simulink model "Position_MPC_Adaptive_InnerLoop"  (R2018a)
settings: Solver=VariableStepAuto  StartTime=0.0  StopTime=inf  RelTol=1e-3
undefined symbols (not defined in the file): Ad, Bd, Beta, C1, C2, cBW, d, Discrete, dw, I, Iw, Kb, Kg, Kt, L, La, mc, md, R, Ra, sampleTime, Time, Waypoint
libraries: mobileRoboticsLib x2, cstblocks x2, mpclib x1, ctrlSharedLib x1, dspsrcs4 x1
settings Model: Creator=shravan  LastModifiedBy=shravan

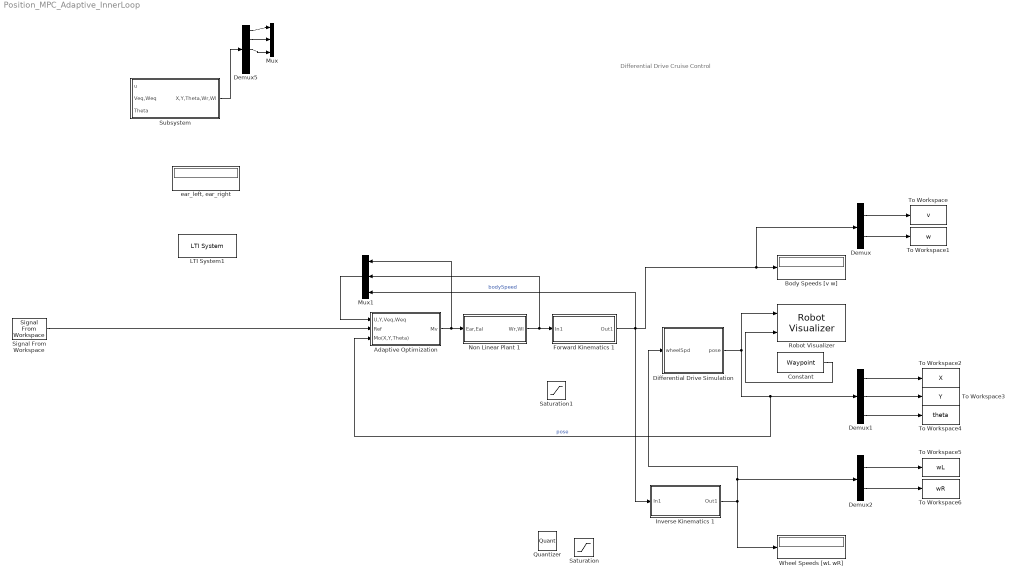
== system Position_MPC_Adaptive_InnerLoop ==
  note: Differential Drive Cruise Control
  "Adaptive Optimization " : Subsystem
  Body Speeds [v w] : Display
  Constant : Constant  Value=Waypoint  SampleTime=sampleTime
  Demux : Demux  Outputs=2
  Demux1 : Demux  Outputs=3
  Demux2 : Demux  Outputs=2
  Demux5 : Demux  Outputs=5
  Differential Drive Simulation : Subsystem  AncestorBlock=mobileRoboticsLib/Kinematic Models/Differential Drive/Differential Drive Simulation  OverrideUsingVariant=mode==2  mask(Differential Drive Simulation){wheelRadius=R, wheelBase=L, initX=C1, initY=C2, initAngle=0, Ts=sampleTime}
      mask prompts: wheelRadius "Wheel Radius [m]"; wheelBase "Wheelbase [m]"; initX "Initial X Position [m]"; initY "Initial Y Position [m]"; initAngle "Initial Angle [rad]"; Ts "Sample Time"
      mask help:
      | Simulates the kinematics of a differential drive vehicle from a specified initial pose.
      |
      | Input: Left and right wheel speeds [wL; wR], in rad/s
      |
      | Output: Pose [x; y; theta], in m, m, and rad
      |
      | Set the Sample Time parameter to 0 for continuous-time simulation, or a positive number for discrete-time simulation.
      mask Help: web('matlab:edit mrsDocDifferentialDrive')
      mask Callback Ts:
      | Ts = evalin('base',get_param(gcb,'Ts'));
      | blk = [gcb '/Generic Robot Simulation/Velocity Integrator'];
      | if Ts > 0
      |     set_param(blk,'OverrideUsingVariant','mode==2');
      | else
      |     set_param(blk,'OverrideUsingVariant','mode==1');
      | end
  Forward Kinematics 1 : Subsystem
  Inverse Kinematics 1 : Subsystem
  LTI System1 : cstblocks/LTI System  sys=Controller  IC=[]
  Mux : Mux  Inputs=3
  Mux1 : Mux  Inputs=3
  Non Linear Plant 1 : Subsystem
  Quantizer : Quantizer
  Robot Visualizer : mobileRoboticsLib/Environments/Robot Visualizer  Priority=99  robotRadius=1  showTrajectory=on  hasWaypoints=on  hasLidar=off  sensorOffset=[ 0 0 ]  scanAngles=[-pi/4,0,pi/4]  hasObjDetector=off  objDetectorOffset=[ 0, 0 ]  objDetectorAngle=0  objDetectorFOV=pi/4  objDetectorMaxRange=5  objectColors=[ 1, 0, 0; 0, 1, 0; 0, 0, 1 ]  objectMarkers='s'
      settings: SourceProductName=Mobile Robotics Simulation Library
  Saturation : Saturate
  Saturation1 : Saturate  UpperLimit=12  LowerLimit=0
  Signal From Workspace : dspsrcs4/Signal From Workspace  X=Lyapunov  Ts=cBW  nsamps=1  OutputAfterFinalValue=Holding final value  ignoreOrWarnInputAndFrameLengths=off  OutputFrames=off
  Subsystem : Subsystem
  To Workspace : ToWorkspace  VariableName=v  SampleTime=-1
  To Workspace1 : ToWorkspace  VariableName=w  SampleTime=-1
  To Workspace2 : ToWorkspace  VariableName=X  SampleTime=sampleTime
  To Workspace3 : ToWorkspace  VariableName=Y  SampleTime=-1
  To Workspace4 : ToWorkspace  VariableName=theta  SampleTime=-1
  To Workspace5 : ToWorkspace  VariableName=wL  SampleTime=-1
  To Workspace6 : ToWorkspace  VariableName=wR  SampleTime=-1
  Wheel Speeds [wL wR] : Display
  "ear_left, ear_right " : Display
  wires:
  Demux5/2 -> Mux/2
  Subsystem/1(X,Y,Theta,Wr,Wl) -> Demux5/1
  Demux5/1 -> Mux/1
  Demux5/3 -> Mux/3
  Inverse Kinematics 1/1(Out1) -> Differential Drive Simulation/1(wheelSpd), Demux2/1, Wheel Speeds [wL wR]/1
  Demux2/2 -> To Workspace6/1
  Demux1/3 -> To Workspace4/1
  Demux1/2 -> To Workspace3/1
  Demux/1 -> To Workspace/1
  Demux/2 -> To Workspace1/1
  "Adaptive Optimization "/1(Mv) -> Non Linear Plant 1/1("Ear,Eal "), Mux1/1
  Differential Drive Simulation/1(pose) -> "Adaptive Optimization "/3(Mo(X,Y,Theta)), Demux1/1, Robot Visualizer/1  "pose"
  Non Linear Plant 1/1(Wr,Wl) -> Mux1/2, Forward Kinematics 1/1(In1)
  Demux1/1 -> To Workspace2/1
  Mux1/1 -> "Adaptive Optimization "/1(U,Y,Veq,Weq)
  Demux2/1 -> To Workspace5/1
  Constant/1 -> Robot Visualizer/2
  Forward Kinematics 1/1(Out1) -> Mux1/3, Inverse Kinematics 1/1(In1), Demux/1, Body Speeds [v w]/1  "bodySpeed"
  Signal From Workspace/1 -> "Adaptive Optimization "/2(Ref)

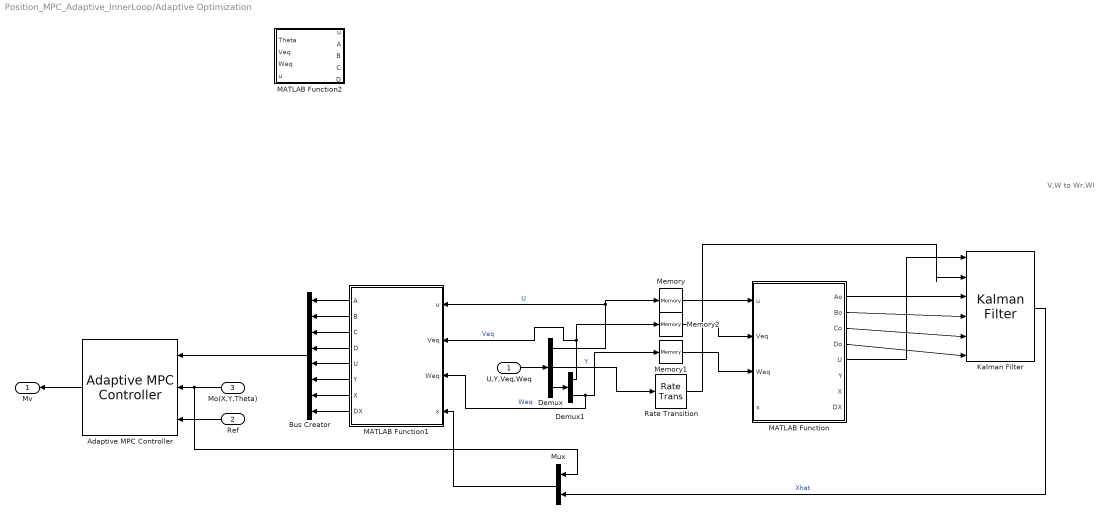
== system Position_MPC_Adaptive_InnerLoop/Adaptive Optimization  ==
  note: V,W to Wr,Wl
  U,Y,Veq,Weq : Inport
  Ref : Inport  Port=2
  Mo(X,Y,Theta) : Inport  Port=3
  Adaptive MPC Controller : mpclib/Adaptive MPC Controller  SCDEnableBlockLinearizationSpecification=on  mpcobj=mpc_pos  updateMPCinCallerWorkspace=on  md_inport=off  mv_inport=off  cost_outport=off  return_sequence=off  return_qpstatus=off  return_state=off  state_inport=off  isltv_plant=off  lims_inport=off  cc_inport=off  ywt_inport=off  uwt_inport=off  duwt_inport=off  rhoeps_inport=off  uref_inport=off  BlockDataType=double  SampleTimeInherited=off  switch_inport=off
      settings: SourceProductName=Model Predictive Control Toolbox
  Bus Creator : BusCreator  Inputs=8
  Demux : Demux  Outputs=3
  Demux1 : Demux  Outputs=2
  Kalman Filter : ctrlSharedLib/Kalman Filter  TimeDomain=Discrete-Time  UseCurrentEstimator=on  ModelSource=Input port  ModelSourceVariable=Plant  A=0.95  B=1  C=1  D=0  NumberOfStates=4  NumberOfInputs=2  NumberOfOutputs=2  InitialEstimateSource=Dialog  X0=0  P0=0.1  UseK=off  UseGH=off  NumberOfProcessNoiseInputs=1  G=1  TimeInvariantG=on  H=0  TimeInvariantH=on  Q=diag([100 100 100 100])  TimeInvariantQ=on  R=diag([0.0001 0.0001])  TimeInvariantR=on  N=0  TimeInvariantN=on  AddInputPort=on  AddEnablePort=off  OutputEstimatedY=off  OutputP=off  Ts=sampleTime
      settings: SourceProductBaseCode=CT
  MATLAB Function : MATLAB Function  TreatAsAtomicUnit=on  SystemSampleTime=sampleTime
  MATLAB Function1 : MATLAB Function  TreatAsAtomicUnit=on  SystemSampleTime=sampleTime
  MATLAB Function2 : MATLAB Function  TreatAsAtomicUnit=on  SystemSampleTime=sampleTime*0.1
  Memory : Memory
  Memory1 : Memory
  Memory2 : Memory
  Mux : Mux  Inputs=2
  Rate Transition : RateTransition  OutPortSampleTime=sampleTime
  Mv : Outport
  wires:
  U,Y,Veq,Weq/1 -> Demux/1
  Memory/1 -> MATLAB Function/1(u)
  Demux/1 -> Memory/1, MATLAB Function1/1(u)  "U"
  Memory2/1 -> MATLAB Function/2(Veq)
  Memory1/1 -> MATLAB Function/3(Weq)
  MATLAB Function/1(Ao) -> Kalman Filter/3
  MATLAB Function/2(Bo) -> Kalman Filter/4
  MATLAB Function/3(Co) -> Kalman Filter/5
  MATLAB Function/4(Do) -> Kalman Filter/6
  MATLAB Function/5(U) -> Kalman Filter/1
  Demux/2 -> Rate Transition/1  "Y"
  Rate Transition/1 -> Kalman Filter/2
  MATLAB Function1/1(A) -> Bus Creator/1
  MATLAB Function1/2(B) -> Bus Creator/2
  MATLAB Function1/3(C) -> Bus Creator/3
  MATLAB Function1/4(D) -> Bus Creator/4
  MATLAB Function1/5(U) -> Bus Creator/5
  MATLAB Function1/6(Y) -> Bus Creator/6
  MATLAB Function1/7(X) -> Bus Creator/7
  MATLAB Function1/8(DX) -> Bus Creator/8
  Bus Creator/1 -> Adaptive MPC Controller/1
  Mo(X,Y,Theta)/1 -> Mux/1, Adaptive MPC Controller/2
  Ref/1 -> Adaptive MPC Controller/3
  Adaptive MPC Controller/1 -> Mv/1
  Demux/3 -> Demux1/1
  Demux1/1 -> MATLAB Function1/2(Veq), Memory2/1  "Veq"
  Demux1/2 -> MATLAB Function1/3(Weq), Memory1/1  "Weq"
  Kalman Filter/1 -> Mux/2  "Xhat"
  Mux/1 -> MATLAB Function1/4(x)

== system Position_MPC_Adaptive_InnerLoop/Differential Drive Simulation ==
  wheelSpd : Inport
  Constant : Constant  Value=0
  Demux : Demux  Outputs=2
  Forward Kinematics 1 : Subsystem
  Generic Robot Simulation : mobileRoboticsLib/Utilities/Generic Vehicle Simulation  initX=initX  initY=initY  initAngle=initAngle  Ts=Ts
      link override Velocity Integrator: OverrideUsingVariant=mode==2
      settings: SourceProductName=Mobile Robotics Simulation Toolbox
  Mux1 : Mux  Inputs=3
  pose : Outport
  wires:
  Generic Robot Simulation/1 -> pose/1
  Forward Kinematics 1/1(Out1) -> Demux/1
  wheelSpd/1 -> Forward Kinematics 1/1(In1)
  Constant/1 -> Mux1/2  "vy"
  Demux/2 -> Mux1/3  "w"
  Demux/1 -> Mux1/1  "vx"
  Mux1/1 -> Generic Robot Simulation/1

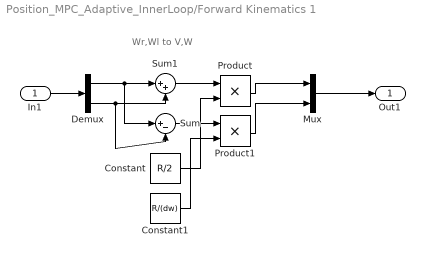
== system Position_MPC_Adaptive_InnerLoop/Forward Kinematics 1 ==
  note: Wr,Wl to V,W
  In1 : Inport
  Constant : Constant  Value=R/2
  Constant1 : Constant  Value=R/(dw)
  Demux : Demux  Outputs=2
  Mux : Mux  Inputs=2
  Product : Product
  Product1 : Product
  Sum : Sum  Inputs=|+-
  Sum1 : Sum  Inputs=|++
  Out1 : Outport
  wires:
  In1/1 -> Demux/1
  Product1/1 -> Mux/2
  Mux/1 -> Out1/1
  Product/1 -> Mux/1
  Demux/1 -> Sum/1, Sum1/1
  Demux/2 -> Sum/2, Sum1/2
  Sum1/1 -> Product/1
  Constant/1 -> Product/2
  Sum/1 -> Product1/1
  Constant1/1 -> Product1/2

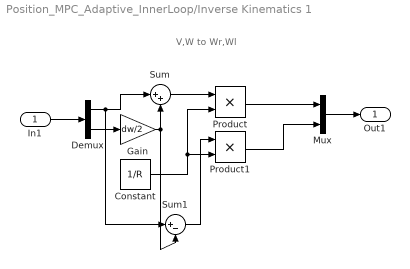
== system Position_MPC_Adaptive_InnerLoop/Inverse Kinematics 1 ==
  note: V,W to Wr,Wl
  In1 : Inport
  Constant : Constant  Value=1/R
  Demux : Demux  Outputs=2
  Gain : Gain  Gain=dw/2
  Mux : Mux  Inputs=2
  Product : Product
  Product1 : Product
  Sum : Sum  Inputs=|++
  Sum1 : Sum  Inputs=|+-
  Out1 : Outport
  wires:
  Gain/1 -> Sum/2, Sum1/2
  Product1/1 -> Mux/2
  Product/1 -> Mux/1
  Sum1/1 -> Product1/1
  Constant/1 -> Product/2, Product1/2
  Sum/1 -> Product/1
  Demux/1 -> Sum/1, Sum1/1
  Demux/2 -> Gain/1
  In1/1 -> Demux/1
  Mux/1 -> Out1/1

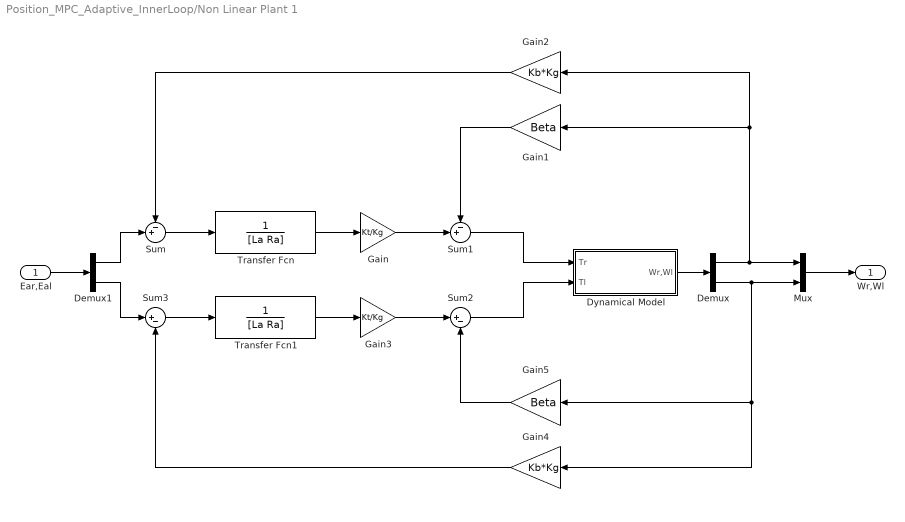
== system Position_MPC_Adaptive_InnerLoop/Non Linear Plant 1 ==
  "Ear,Eal " : Inport
  Demux : Demux  Outputs=2
  Demux1 : Demux  Outputs=2
  Dynamical Model : Subsystem
  Gain : Gain  Gain=Kt/Kg
  Gain1 : Gain  Gain=Beta
  Gain2 : Gain  Gain=Kb*Kg
  Gain3 : Gain  Gain=Kt/Kg
  Gain4 : Gain  Gain=Kb*Kg
  Gain5 : Gain  Gain=Beta
  Mux : Mux  Inputs=2
  Sum : Sum  Inputs=-+|
  Sum1 : Sum  Inputs=-+|
  Sum2 : Sum  Inputs=|+-
  Sum3 : Sum  Inputs=|+-
  Transfer Fcn : TransferFcn  Denominator=[La Ra]
  Transfer Fcn1 : TransferFcn  Denominator=[La Ra]
  Wr,Wl : Outport
  wires:
  Sum2/1 -> Dynamical Model/2(Tl)
  Demux/2 -> Mux/2, Gain5/1, Gain4/1
  Gain3/1 -> Sum2/1
  Transfer Fcn1/1 -> Gain3/1
  Transfer Fcn/1 -> Gain/1
  Sum1/1 -> Dynamical Model/1(Tr)
  "Ear,Eal "/1 -> Demux1/1
  Gain/1 -> Sum1/2
  Gain2/1 -> Sum/1
  Mux/1 -> Wr,Wl/1
  Sum3/1 -> Transfer Fcn1/1
  Demux1/1 -> Sum/2
  Dynamical Model/1(Wr,Wl) -> Demux/1
  Demux/1 -> Gain1/1, Gain2/1, Mux/1
  Gain1/1 -> Sum1/1
  Demux1/2 -> Sum3/1
  Sum/1 -> Transfer Fcn/1
  Gain4/1 -> Sum3/2
  Gain5/1 -> Sum2/2

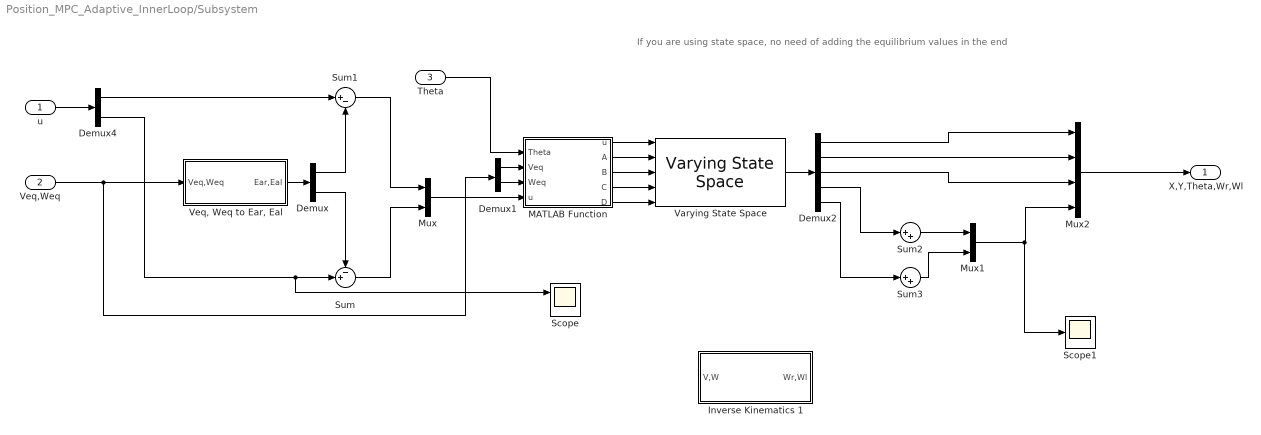
== system Position_MPC_Adaptive_InnerLoop/Subsystem ==
  note: If you are using state space, no need of adding the equilibrium values in the end
  "u " : Inport
  "Veq,Weq " : Inport  Port=2
  "Theta " : Inport  Port=3
  Demux : Demux  Outputs=2
  Demux1 : Demux  Outputs=2
  Demux2 : Demux  Outputs=5
  Demux4 : Demux  Outputs=2
  Inverse Kinematics 1 : Subsystem
  MATLAB Function : MATLAB Function  TreatAsAtomicUnit=on  SystemSampleTime=sampleTime*0.1
  Mux : Mux  Inputs=2
  Mux1 : Mux  Inputs=2
  Mux2 : Mux
  Scope : Scope  NumInputPorts=2
  Scope1 : Scope
  Sum : Sum  Inputs=-+|
  Sum1 : Sum  Inputs=|+-
  Sum2 : Sum  Inputs=|++
  Sum3 : Sum  Inputs=|++
  Varying State Space : cstblocks/Linear Parameter Varying/Varying State Space  x0=[C1;C2;0;0;0;0;0]  xNames=''  OutputX=off  OutputDX=off
      settings: SourceProductName=Control System Toolbox
  "Veq, Weq to Ear, Eal " : Subsystem
  X,Y,Theta,Wr,Wl : Outport
  wires:
  "Veq, Weq to Ear, Eal "/1(Ear,Eal) -> Demux/1
  Demux/1 -> Sum1/2
  Demux/2 -> Sum/1
  MATLAB Function/3(B) -> Varying State Space/3
  MATLAB Function/4(C) -> Varying State Space/4
  MATLAB Function/1(u) -> Varying State Space/1
  MATLAB Function/2(A) -> Varying State Space/2
  MATLAB Function/5(D) -> Varying State Space/5
  Sum1/1 -> Mux/1
  Sum/1 -> Mux/2
  Mux/1 -> MATLAB Function/4("u ")
  "Theta "/1 -> MATLAB Function/1(Theta)
  Demux1/2 -> MATLAB Function/3(Weq)
  Demux1/1 -> MATLAB Function/2(Veq)
  Varying State Space/1 -> Demux2/1
  Demux2/1 -> Mux2/1
  Demux2/2 -> Mux2/2
  Demux2/3 -> Mux2/3
  Demux2/4 -> Sum2/1
  Demux2/5 -> Sum3/1
  Mux1/1 -> Scope1/1, Mux2/4
  Sum2/1 -> Mux1/1
  Sum3/1 -> Mux1/2
  "Veq,Weq "/1 -> "Veq, Weq to Ear, Eal "/1(Veq,Weq), Demux1/1
  Mux2/1 -> X,Y,Theta,Wr,Wl/1
  "u "/1 -> Demux4/1
  Demux4/1 -> Sum1/1
  Demux4/2 -> Scope/1, Sum/2

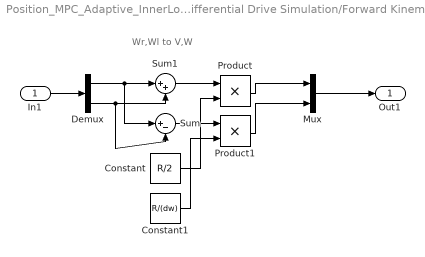
== system Position_MPC_Adaptive_InnerLoop/Differential Drive Simulation/Forward Kinematics 1 ==
  note: Wr,Wl to V,W
  In1 : Inport
  Constant : Constant  Value=R/2
  Constant1 : Constant  Value=R/(dw)
  Demux : Demux  Outputs=2
  Mux : Mux  Inputs=2
  Product : Product
  Product1 : Product
  Sum : Sum  Inputs=|+-
  Sum1 : Sum  Inputs=|++
  Out1 : Outport
  wires:
  In1/1 -> Demux/1
  Product1/1 -> Mux/2
  Mux/1 -> Out1/1
  Product/1 -> Mux/1
  Demux/1 -> Sum/1, Sum1/1
  Demux/2 -> Sum/2, Sum1/2
  Sum1/1 -> Product/1
  Constant/1 -> Product/2
  Sum/1 -> Product1/1
  Constant1/1 -> Product1/2

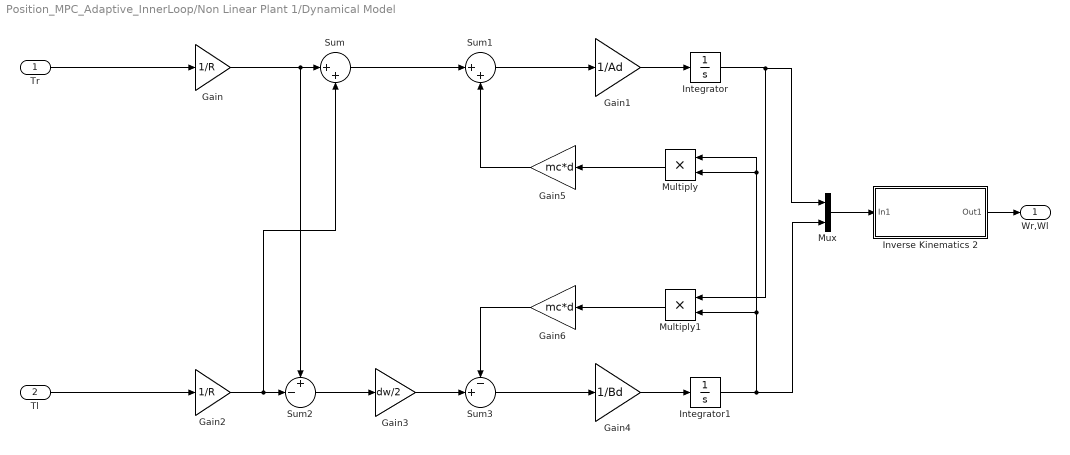
== system Position_MPC_Adaptive_InnerLoop/Non Linear Plant 1/Dynamical Model ==
  Tr : Inport
  Tl : Inport  Port=2
  Gain : Gain  Gain=1/R
  Gain1 : Gain  Gain=1/Ad
  Gain2 : Gain  Gain=1/R
  Gain3 : Gain  Gain=dw/2
  Gain4 : Gain  Gain=1/Bd
  Gain5 : Gain  Gain=mc*d
  Gain6 : Gain  Gain=mc*d
  Integrator : Integrator
  Integrator1 : Integrator
  Inverse Kinematics 2 : Subsystem
  Multiply : Product
  Multiply1 : Product
  Mux : Mux  Inputs=2
  Sum : Sum  Inputs=|++
  Sum1 : Sum  Inputs=|++
  Sum2 : Sum  Inputs=+-|
  Sum3 : Sum  Inputs=-+|
  Wr,Wl : Outport
  wires:
  Gain1/1 -> Integrator/1
  Tl/1 -> Gain2/1
  Gain6/1 -> Sum3/1
  Gain2/1 -> Sum2/2, Sum/2
  Sum2/1 -> Gain3/1
  Gain3/1 -> Sum3/2
  Multiply/1 -> Gain5/1
  Integrator1/1 -> Mux/2, Multiply/1, Multiply/2, Multiply1/2
  Tr/1 -> Gain/1
  Gain5/1 -> Sum1/2
  Sum/1 -> Sum1/1
  Inverse Kinematics 2/1(Out1) -> Wr,Wl/1
  Gain4/1 -> Integrator1/1
  Mux/1 -> Inverse Kinematics 2/1(In1)
  Integrator/1 -> Multiply1/1, Mux/1
  Gain/1 -> Sum2/1, Sum/1
  Sum3/1 -> Gain4/1
  Multiply1/1 -> Gain6/1
  Sum1/1 -> Gain1/1

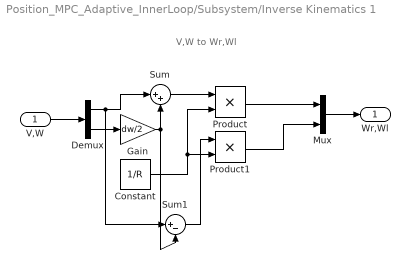
== system Position_MPC_Adaptive_InnerLoop/Subsystem/Inverse Kinematics 1 ==
  note: V,W to Wr,Wl
  V,W : Inport
  Constant : Constant  Value=1/R
  Demux : Demux  Outputs=2
  Gain : Gain  Gain=dw/2
  Mux : Mux  Inputs=2
  Product : Product
  Product1 : Product
  Sum : Sum  Inputs=|++
  Sum1 : Sum  Inputs=|+-
  Wr,Wl : Outport
  wires:
  Gain/1 -> Sum/2, Sum1/2
  Product1/1 -> Mux/2
  Product/1 -> Mux/1
  Sum1/1 -> Product1/1
  Constant/1 -> Product/2, Product1/2
  Sum/1 -> Product/1
  Demux/1 -> Sum/1, Sum1/1
  Demux/2 -> Gain/1
  V,W/1 -> Demux/1
  Mux/1 -> Wr,Wl/1

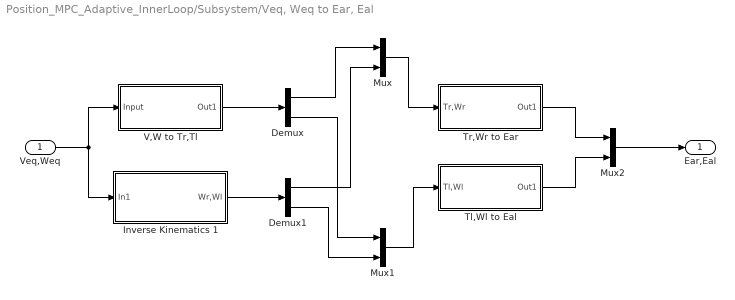
== system Position_MPC_Adaptive_InnerLoop/Subsystem/Veq, Weq to Ear, Eal  ==
  Veq,Weq : Inport
  Demux : Demux  Outputs=2
  Demux1 : Demux  Outputs=2
  Inverse Kinematics 1 : Subsystem
  Mux : Mux  Inputs=2
  Mux1 : Mux  Inputs=2
  Mux2 : Mux  Inputs=2
  Tl,Wl to Eal : Subsystem
  Tr,Wr to Ear : Subsystem
  V,W to Tr,Tl : Subsystem
  Ear,Eal : Outport
  wires:
  V,W to Tr,Tl/1(Out1) -> Demux/1
  Demux/1 -> Mux/1
  Mux/1 -> Tr,Wr to Ear/1(Tr,Wr)
  Veq,Weq/1 -> Inverse Kinematics 1/1(In1), V,W to Tr,Tl/1(Input)
  Inverse Kinematics 1/1(Wr,Wl) -> Demux1/1
  Demux1/1 -> Mux/2
  Demux/2 -> Mux1/1
  Demux1/2 -> Mux1/2
  Mux1/1 -> Tl,Wl to Eal/1(Tl,Wl)
  Tr,Wr to Ear/1(Out1) -> Mux2/1
  Tl,Wl to Eal/1(Out1) -> Mux2/2
  Mux2/1 -> Ear,Eal/1

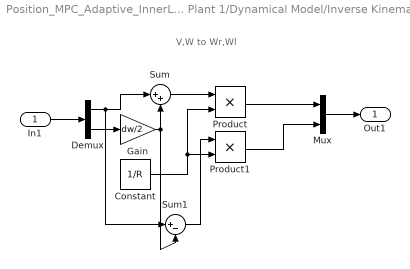
== system Position_MPC_Adaptive_InnerLoop/Non Linear Plant 1/Dynamical Model/Inverse Kinematics 2 ==
  note: V,W to Wr,Wl
  In1 : Inport
  Constant : Constant  Value=1/R
  Demux : Demux  Outputs=2
  Gain : Gain  Gain=dw/2
  Mux : Mux  Inputs=2
  Product : Product
  Product1 : Product
  Sum : Sum  Inputs=|++
  Sum1 : Sum  Inputs=|+-
  Out1 : Outport
  wires:
  Product1/1 -> Mux/2
  Product/1 -> Mux/1
  Sum1/1 -> Product1/1
  Constant/1 -> Product/2, Product1/2
  Sum/1 -> Product/1
  Gain/1 -> Sum/2, Sum1/2
  Demux/1 -> Sum/1, Sum1/1
  Demux/2 -> Gain/1
  In1/1 -> Demux/1
  Mux/1 -> Out1/1

== system Position_MPC_Adaptive_InnerLoop/Subsystem/Veq, Weq to Ear, Eal /Inverse Kinematics 1 ==
  note: V,W to Wr,Wl
  In1 : Inport
  Constant : Constant  Value=1/R
  Demux : Demux  Outputs=2
  Gain : Gain  Gain=dw/2
  Mux : Mux  Inputs=2
  Product : Product
  Product1 : Product
  Sum : Sum  Inputs=|++
  Sum1 : Sum  Inputs=|+-
  Wr,Wl : Outport
  wires:
  Mux/1 -> Wr,Wl/1
  In1/1 -> Demux/1
  Demux/2 -> Gain/1
  Demux/1 -> Sum1/1, Sum/1
  Sum/1 -> Product/1
  Constant/1 -> Product1/2, Product/2
  Sum1/1 -> Product1/1
  Product/1 -> Mux/1
  Product1/1 -> Mux/2
  Gain/1 -> Sum1/2, Sum/2

== system Position_MPC_Adaptive_InnerLoop/Subsystem/Veq, Weq to Ear, Eal /Tl,Wl to Eal ==
  Tl,Wl : Inport
  Demux1 : Demux  Outputs=2
  Gain : Gain  Gain=Ra*Kg/Kt
  Gain1 : Gain  Gain=Beta
  Gain2 : Gain  Gain=Ra*Kg/Kt
  Gain3 : Gain  Gain=Kb*Kg
  Sum : Sum  Inputs=|+++
  Out1 : Outport
  wires:
  Gain1/1 -> Sum/2
  Gain2/1 -> Gain1/1
  Gain/1 -> Sum/1
  Gain3/1 -> Sum/3
  Sum/1 -> Out1/1
  Tl,Wl/1 -> Demux1/1
  Demux1/1 -> Gain/1
  Demux1/2 -> Gain3/1, Gain2/1

== system Position_MPC_Adaptive_InnerLoop/Subsystem/Veq, Weq to Ear, Eal /Tr,Wr to Ear ==
  Tr,Wr : Inport
  Demux1 : Demux  Outputs=2
  Gain : Gain  Gain=Ra*Kg/Kt
  Gain1 : Gain  Gain=Beta
  Gain2 : Gain  Gain=Ra*Kg/Kt
  Gain3 : Gain  Gain=Kb*Kg
  Sum : Sum  Inputs=|+++
  Out1 : Outport
  wires:
  Gain2/1 -> Gain1/1
  Tr,Wr/1 -> Demux1/1
  Sum/1 -> Out1/1
  Gain1/1 -> Sum/2
  Gain3/1 -> Sum/3
  Demux1/2 -> Gain3/1, Gain2/1
  Gain/1 -> Sum/1
  Demux1/1 -> Gain/1

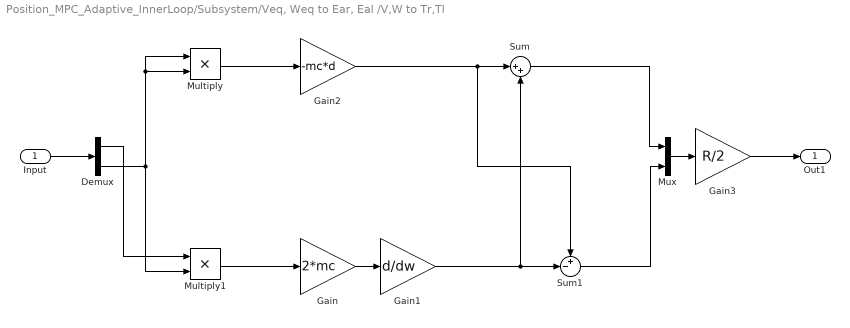
== system Position_MPC_Adaptive_InnerLoop/Subsystem/Veq, Weq to Ear, Eal /V,W to Tr,Tl ==
  Input : Inport
  Demux : Demux  Outputs=2
  Gain : Gain  Gain=2*mc
  Gain1 : Gain  Gain=d/dw
  Gain2 : Gain  Gain=-mc*d
  Gain3 : Gain  Gain=R/2
  Multiply : Product
  Multiply1 : Product
  Mux : Mux  Inputs=2
  Sum : Sum  Inputs=|++
  Sum1 : Sum  Inputs=+-|
  Out1 : Outport
  wires:
  Demux/1 -> Multiply1/1
  Mux/1 -> Gain3/1
  Gain/1 -> Gain1/1
  Input/1 -> Demux/1
  Multiply1/1 -> Gain/1
  Sum1/1 -> Mux/2
  Gain1/1 -> Sum1/2, Sum/2
  Gain2/1 -> Sum1/1, Sum/1
  Demux/2 -> Multiply1/2, Multiply/2, Multiply/1
  Gain3/1 -> Out1/1
  Multiply/1 -> Gain2/1
  Sum/1 -> Mux/1

== matlab function Position_MPC_Adaptive_InnerLoop/Adaptive Optimization /MATLAB Function2 ==
  data: Theta input size=[1,1]; Veq input size=[1,1]; Weq input size=[1,1]; u input size=[2,1]; u output; A output; B output; C output; D output; sampleTime parameter; I parameter; Iw parameter; R parameter
function [u,A,B,C,D] = fcn(Theta,Veq,Weq,u,sampleTime,I, Iw,R)
% Sample time
Ts = sampleTime;
d = 0.0107; L = 0.28; AR = L/0.25; dw = 0.25; md = 0;
d = 0; thetaeq = Theta;
% Model Parameters
Kt = 0.0046; Kg = 50; Kb = Kt; Beta = 2.29e-06; La =1.729e-03; Ra = 5.51;
m = 3.4; mc = 2.76 + md; I = I ; Iw = Iw; L = L; d = d; dw = dw; 
Ao = m + 2*Iw/(R*R); Bo = I + dw*dw*Iw/(2*R*R);

% Continuous-time model for Plant e_r, e_l to Wr,Wl
% ULTIMATE - CORRECT representation of Plant using State Space form derived
% on Aug 24 th, 2020 
Ac = [-2*Beta/(Ao*R*R) 2*mc*d*Weq/Ao   (Kt/(Kg*R*Ao))  (Kt/(Kg*R*Ao));
     -mc*d*Weq/Bo  (-mc*d*Veq/Bo)-(Beta*dw*dw/(2*R*R*Bo)) dw*Kt/(2*Kg*R*Bo) -dw*Kt/(2*Kg*Bo*R) ;
     -Kb*Kg/(La*R)   -Kb*Kg*dw/(2*La*R)  -Ra/La      0 ;
     -Kb*Kg/(La*R)    Kb*Kg*dw/(2*La*R)    0       -Ra/La ];
Bc = [0 0; 0 0; 1/La 0; 0 1/La]; Cc =  [1/R dw/(2*R); 1/R -dw/(2*R)]*[1 0 0 0; 0 1 0 0]; Dc = [0 0;0 0];


% States x,y,theta, V,W, Iar,Ial 

Au =      [0  0  -Veq*sin(thetaeq) cos(thetaeq)  0  0  0;
           0  0  Veq*cos(thetaeq) sin(thetaeq)  0  0  0;
           0  0  0                 0            1  0  0;  
           zeros(4,3) Ac]
Bu =      [0 0;
           0 0;
           0 0;
           Bc]
Cu =      [1 0 0 0 0 0 0;
           0 1 0 0 0 0 0;
           0 0 1 0 0 0 0;
           zeros(2,3) Cc]
Du =       zeros(5,2)

% Discretize the continuous-time model using zero-order hold 
% on the inputs and a sample time of Ts seconds
nx = size(Au,1);
nu = size(Bu,2);
M = expm([[Au Bu]*Ts; zeros(nu,nx+nu)]);
A = Au;%M(1:nx,1:nx);
B = Bu;%M(1:nx,nx+1:nx+nu);
C = Cu;
D = Du;

% Nominal conditions for discrete-time plant
%X = x;
u = u;
%Y = Co*x + Do*u;
%DX = Ao*x+Bo*u-x;
%y = u;

== matlab function Position_MPC_Adaptive_InnerLoop/Subsystem/MATLAB Function ==
  data: Theta input size=[1,1]; Veq input size=[1,1]; Weq input size=[1,1]; u input size=[2,1]; u output; A output; B output; C output; D output; sampleTime parameter; I parameter; Iw parameter; R parameter
function [u,A,B,C,D] = fcn(Theta,Veq,Weq,u,sampleTime,I, Iw,R)
% Sample time
Ts = sampleTime;
d = 0.0107; L = 0.28; AR = L/0.25; dw = 0.25; md = 0;
d = 0; thetaeq = Theta;
% Model Parameters
Kt = 0.0046; Kg = 50; Kb = Kt; Beta = 2.29e-06; La =1.729e-03; Ra = 5.51;
m = 3.4; mc = 2.76 + md; I = I ; Iw = Iw; L = L; d = d; dw = dw; 
Ao = m + 2*Iw/(R*R); Bo = I + dw*dw*Iw/(2*R*R);

% Continuous-time model for Plant e_r, e_l to Wr,Wl
% ULTIMATE - CORRECT representation of Plant using State Space form derived
% on Aug 24 th, 2020 
Ac = [-2*Beta/(Ao*R*R) 2*mc*d*Weq/Ao   (Kt/(Kg*R*Ao))  (Kt/(Kg*R*Ao));
     -mc*d*Weq/Bo  (-mc*d*Veq/Bo)-(Beta*dw*dw/(2*R*R*Bo)) dw*Kt/(2*Kg*R*Bo) -dw*Kt/(2*Kg*Bo*R) ;
     -Kb*Kg/(La*R)   -Kb*Kg*dw/(2*La*R)  -Ra/La      0 ;
     -Kb*Kg/(La*R)    Kb*Kg*dw/(2*La*R)    0       -Ra/La ];
Bc = [0 0; 0 0; 1/La 0; 0 1/La]; Cc =  [1/R dw/(2*R); 1/R -dw/(2*R)]*[1 0 0 0; 0 1 0 0]; Dc = [0 0;0 0];


% States x,y,theta, V,W, Iar,Ial 

Au =      [0  0  -Veq*sin(thetaeq) cos(thetaeq)  0  0  0;
           0  0  Veq*cos(thetaeq) sin(thetaeq)  0  0  0;
           0  0  0                 0            1  0  0;  
           zeros(4,3) Ac]
Bu =      [0 0;
           0 0;
           0 0;
           Bc]
Cu =      [1 0 0 0 0 0 0;
           0 1 0 0 0 0 0;
           0 0 1 0 0 0 0;
           zeros(2,3) Cc]
Du =       zeros(5,2)

% Discretize the continuous-time model using zero-order hold 
% on the inputs and a sample time of Ts seconds
nx = size(Au,1);
nu = size(Bu,2);
M = expm([[Au Bu]*Ts; zeros(nu,nx+nu)]);
A = Au;%M(1:nx,1:nx);
B = Bu;%M(1:nx,nx+1:nx+nu);
C = Cu;
D = Du;

% Nominal conditions for discrete-time plant
%X = x;
u = u;
%Y = Co*x + Do*u;
%DX = Ao*x+Bo*u-x;
%y = u;

== matlab function Position_MPC_Adaptive_InnerLoop/Adaptive Optimization /MATLAB Function ==
  data: u input size=[2,1]; Veq input size=[1,1]; Weq input size=[1,1]; Ao output size=[4,4]; x input size=[4,1]; Bo output size=[4,2]; Co output size=[2,4]; Do output size=[2,2]; U output size=[2,1]; Y output size=[2,1]; X output size=[4,1]; DX output size=[4,1]; sampleTime parameter size=[1,1]; d parameter size=[1,1]; dw parameter size=[1,1]; Iw parameter size=[1,1]; I parameter size=[1,1]; md parameter size=1,1; R parameter size=1,1; L parameter size=1,1
function [Ao,Bo,Co,Do,U,Y,X,DX] = fcn(u,Veq,Weq,x,sampleTime,d, dw, Iw, I, md, R, L)
% Sample time
Ts = sampleTime;

% Model Parameters
Kt = 0.0046; Kg = 50; Kb = Kt; Beta = 2.29e-06; La =1.729e-03; Ra = 5.51;
m = 3.4; mc = 2.76 + md; I = I ; Iw = Iw; L = L; d = d; dw = dw; 
A = m + 2*Iw/(R*R); B = I + dw*dw*Iw/(2*R*R);

% Continuous-time model for Plant e_r, e_l to Wr,Wl
Ac = [-2*Beta*Kg*Kg/(A*R*R)  2*mc*d*Weq/A   (Kt*Kg/(R*A))  (Kt*Kg/(A*R));
      -mc*d*Weq/B  (-mc*d*Veq/B)-(Beta*dw*dw*Kg*Kg/(2*R*R*B)) dw*Kt*Kg/(2*R*B) -dw*Kt*Kg/(2*B*R) ;
     -Kb*Kg/(La*R)   -Kb*Kg*dw/(2*La*R)  -Ra/La      0 ;
     -Kb*Kg/(La*R)    Kb*Kg*dw/(2*La*R)    0       -Ra/La ];
Bc = [0 0; 0 0; 1/La 0; 0 1/La]; Cc =  [1/R dw/(2*R); 1/R -dw/(2*R)]*[1 0 0 0; 0 1 0 0]; Dc = [0 0;0 0];


% Discretize the continuous-time model using zero-order hold 
% on the inputs and a sample time of Ts seconds
nx = size(Ac,1);
nu = size(Bc,2);
M = expm([[Ac Bc]*Ts; zeros(nu,nx+nu)]);
Ao = M(1:nx,1:nx);
Bo = M(1:nx,nx+1:nx+nu);
Co = Cc;
Do = Dc;

% Nominal conditions for discrete-time plant
X = x;
U = u;
Y = Co*x + Do*u;
DX = Ao*x+Bo*u-x;

== matlab function Position_MPC_Adaptive_InnerLoop/Adaptive Optimization /MATLAB Function1 ==
  data: u input size=[2,1]; Veq input size=[1,1]; Weq input size=[1,1]; A output size=[7,7]; x input size=[7,1]; B output size=[7,2]; C output size=[3,7]; D output size=[3,2]; U output size=[2,1]; Y output size=[3,1]; X output size=[7,1]; DX output size=[7,1]; sampleTime parameter size=[1,1]; d parameter size=[1,1]; dw parameter size=[1,1]; Iw parameter size=[1,1]; I parameter size=[1,1]; md parameter size=1,1; R parameter size=1,1; L parameter size=1,1
function [A,B,C,D,U,Y,X,DX] = fcn(u,Veq,Weq,x,sampleTime,d, dw, Iw, I, md, R, L)
% Sample time
Ts = sampleTime;

% Model Parameters
Kt = 0.0046; Kg = 50; Kb = Kt; Beta = 2.29e-06; La =1.729e-03; Ra = 5.51;
m = 3.4; mc = 2.76 + md; I = I ; Iw = Iw; L = L; d = d; dw = dw; 
Ao = m + 2*Iw/(R*R); Bo = I + dw*dw*Iw/(2*R*R);
thetaeq = x(3,1);
% Continuous-time model for Plant e_r, e_l to Wr,Wl
% ULTIMATE - CORRECT representation of Plant using State Space form derived
% on Aug 24 th, 2020 
Ac = [-2*Beta/(Ao*R*R) 2*mc*d*Weq/Ao   (Kt/(Kg*R*Ao))  (Kt/(Kg*R*Ao));
     -mc*d*Weq/Bo  (-mc*d*Veq/Bo)-(Beta*dw*dw/(2*R*R*Bo)) dw*Kt/(2*Kg*R*Bo) -dw*Kt/(2*Kg*Bo*R) ;
     -Kb*Kg/(La*R)   -Kb*Kg*dw/(2*La*R)  -Ra/La      0 ;
     -Kb*Kg/(La*R)    Kb*Kg*dw/(2*La*R)    0       -Ra/La ];
Bc = [0 0; 0 0; 1/La 0; 0 1/La]; Cc =  [1/R dw/(2*R); 1/R -dw/(2*R)]*[1 0 0 0; 0 1 0 0]; Dc = [0 0;0 0];


% States x,y,theta, V,W, Iar,Ial 

Au =      [0  0  -Veq*sin(thetaeq) cos(thetaeq)  0  0  0;
           0  0  Veq*cos(thetaeq) sin(thetaeq)  0  0  0;
           0  0  0                 0            1  0  0;  
           zeros(4,3) Ac]
Bu =      [0 0;
           0 0;
           0 0;
           Bc]
Cu =      [1 0 0 0 0 0 0;
           0 1 0 0 0 0 0;
           0 0 1 0 0 0 0]
Du =       zeros(3,2)

% Discretize the continuous-time model using zero-order hold 
% on the inputs and a sample time of Ts seconds
nx = size(Au,1);
nu = size(Bu,2);
M = expm([[Au Bu]*Ts; zeros(nu,nx+nu)]);
A = M(1:nx,1:nx);
B = M(1:nx,nx+1:nx+nu);
C = Cu;
D = Du;

% Nominal conditions for discrete-time plant
X = x;
U = u;
Y = C*x + D*u;
DX = A*x+B*u-x;
